simulink model "pid_subsystem"  (R2023a)
settings: Solver=VariableStepAuto  StartTime=0.0  StopTime=500  RelTol=1e-3
settings Model: Creator=Garv Gupta  LastModifiedBy=Garv Gupta

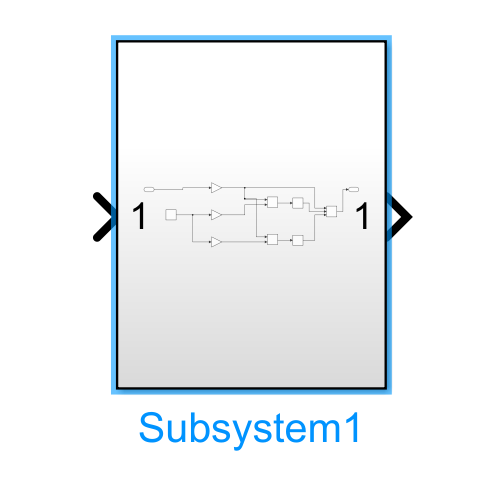
[thumbnail: Simulink's stored preview of the top-level diagram]
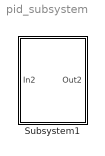
== system pid_subsystem ==
  Subsystem1 : Subsystem

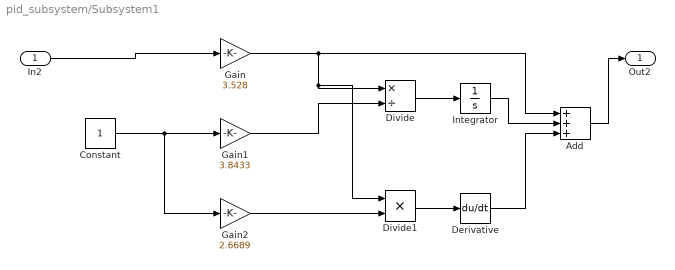
== system pid_subsystem/Subsystem1 ==
  In2 : Inport
  Add : Sum  Inputs=+++
  Constant : Constant
  Derivative : Derivative
  Divide : Product  Inputs=*/
  Divide1 : Product  Inputs=**
  Gain : Gain  Gain=3.528
  Gain1 : Gain  Gain=3.8433
  Gain2 : Gain  Gain=2.6689
  Integrator : Integrator
  Out2 : Outport
  wires:
  In2/1 -> Gain/1
  Gain1/1 -> Divide/2
  Gain2/1 -> Divide1/2
  Gain/1 -> Add/1, Divide1/1, Divide/1
  Constant/1 -> Gain2/1, Gain1/1
  Divide/1 -> Integrator/1
  Divide1/1 -> Derivative/1
  Integrator/1 -> Add/2
  Derivative/1 -> Add/3
  Add/1 -> Out2/1
